simulink model "stateflow1"  (R2013b)
settings: Solver=ode45  StartTime=0.0  StopTime=inf  RelTol=1e-3
settings Model: Creator=daniw  LastModifiedBy=daniw

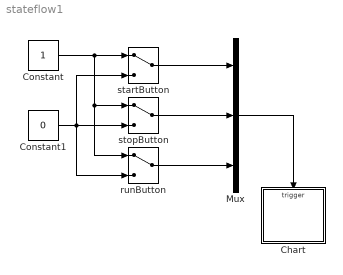
== system stateflow1 ==
  Chart : Stateflow chart  TreatAsAtomicUnit=on
  Constant : Constant
  Constant1 : Constant  Value=0
  Mux : Mux  Inputs=3
  runButton : ManualSwitch
  startButton : ManualSwitch
  stopButton : ManualSwitch
  wires:
  Mux/1 -> Chart/Trigger
  Constant/1 -> runButton/1, stopButton/1, startButton/1
  Constant1/1 -> runButton/2, startButton/2, stopButton/2
  startButton/1 -> Mux/1
  stopButton/1 -> Mux/2
  runButton/1 -> Mux/3

== stateflow chart stateflow1/Chart ==
  state Init
  state Wait
  state Move
  (default) -> Init
  Move -> Init : stopButtonPressed
  Init -> Wait : startButtonPressed
  Wait -> Move : runButtonPressed
  events: startButtonPressed input RISING_EDGE_EVENT; stopButtonPressed input RISING_EDGE_EVENT; runButtonPressed input RISING_EDGE_EVENT
